simulink subsystem "System_Measurement_Vehicle"  (R2023b)
settings: Solver=VariableStepAuto  StartTime=0.0  StopTime=10.0  RelTol=1e-3
settings Model: Creator=20155555  LastModifiedBy=20155555

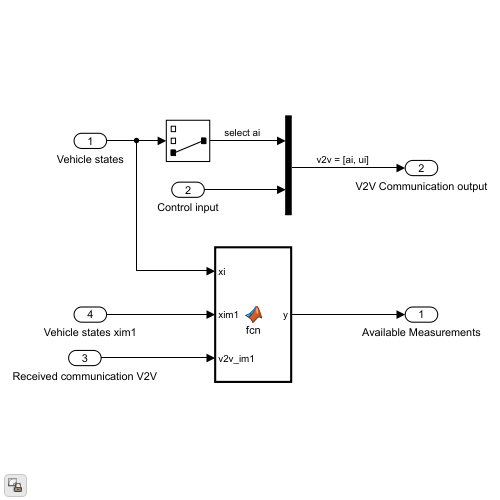
[thumbnail: Simulink's stored preview of the top-level diagram]
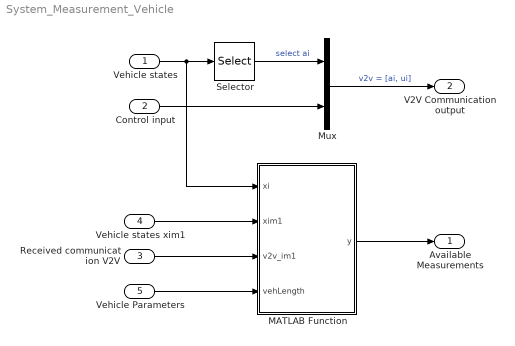
== system System_Measurement_Vehicle ==
  Vehicle states : Inport
  Control input : Inport  Port=2
  Received communication V2V : Inport  Port=3
  Vehicle states xim1 : Inport  Port=4
  Vehicle Parameters : Inport  Port=5
  MATLAB Function : MATLAB Function  TreatAsAtomicUnit=on
  Mux : Mux  Inputs=2
  Selector : Selector  InputPortWidth=3  IndexOptions=Index vector (dialog)  Indices=[3]  OutputSizes=1
  Available Measurements : Outport
  V2V Communication output : Outport  Port=2
  wires:
  Mux/1 -> V2V Communication output/1  "v2v = [ai, ui]"
  Vehicle states/1 -> Selector/1, MATLAB Function/1(xi)
  MATLAB Function/1(y) -> Available Measurements/1
  Received communication V2V/1 -> MATLAB Function/3(v2v_im1)
  Vehicle states xim1/1 -> MATLAB Function/2(xim1)
  Selector/1 -> Mux/1  "select ai"
  Control input/1 -> Mux/2
  Vehicle Parameters/1 -> MATLAB Function/4(vehLength)

== matlab function System_Measurement_Vehicle/MATLAB Function ==
  data: xi input; y output; xim1 input; v2v_im1 input; vehLength input
 function y = fcn(xi, xim1, v2v_im1, vehLength)

% y = [di, vi, ai, vim1-vi, ai, uim1]
% output y = [qim1-qi-L, vi, ai, vim1-vi, ai, uim1

y = [(xim1(1)-xi(1))-vehLength; xi(2:3); xim1(2)-xi(2); v2v_im1];
